simulink model "FAST_RL_Env"  (R2023a)
settings: Solver=FixedStepAuto  StartTime=0.0  StopTime=inf  FixedStep=DT  MaxStep=DT  RelTol=1e-3  EnableMultiTasking=on
undefined symbols (not defined in the file): Cmoment, Cpitch, MaxMoment, Penalty
libraries: rllib x1
settings Model: Creator=bjonkman  LastModifiedBy=Admin
settings SolverCC: AlgebraicLoopSolver=TrustRegion  AutoInsertRateTranBlk=on
settings DataIOCC: LimitDataPoints=on  SaveFormat=Array  SignalLoggingSaveFormat=ModelDataLogs  SaveOutput=off  SaveTime=off  SignalLoggingName=sigsOut
settings OptimizationCC: ReuseModelBlockBuffer=off  ExpressionDepthLimit=2147483647  LifeSpan=inf
settings DebuggingCC: SaveWithParameterizedLinksMsg=none  UnderspecifiedInitializationDetection=Classic  MergeDetectMultiDrivingBlocksExec=none  SignalResolutionControl=TryResolveAllWithWarning  MultiTaskDSMMsg=warning  MultiTaskCondExecSysMsg=none  FcnCallInpInsideContextMsg=warning  UnconnectedInputMsg=warning  UnconnectedOutputMsg=warning  UnconnectedLineMsg=warning  StateNameClashWarn=warning  SFUnexpectedBacktrackingDiag=warning  SFNoUnconditionalDefaultTransitionDiag=warning  SFExecutionAtInitializationDiag=none  ArithmeticOperatorsInVariantConditions=warning
settings HardwareCC: ProdBitPerPointer=32  ProdBitPerSizeT=32  ProdBitPerPtrDiffT=32  ProdLargestAtomicFloat=None  ProdIntDivRoundTo=Undefined  ProdEndianess=Unspecified  ProdWordSize=32  ProdHWDeviceType=32-bit Generic  TargetUnknown=on
settings ModelReferenceCC: EnableRefExpFcnMdlSchedulingChecks=on  PropagateSignalLabelsOutOfModel=off
settings SFSimCC: SimUseLocalCustomCode=off  CustomCodeUndefinedFunction=UseInterfaceOnly
settings RTWCC: RTWUseLocalCustomCode=off  DLArmComputeVersion=19.05
settings CodeAppCC: StateflowObjectComments=on
settings GRTTargetCC: TargetLangStandard=C89/C90 (ANSI)  CombineOutputUpdateFcns=off  GRTInterface=on
settings ConfigComp: CovMetricSettings=dw  CovSaveCumulativeToWorkspaceVar=on  CovSaveSingleToWorkspaceVar=on  CovExternalEMLEnable=off

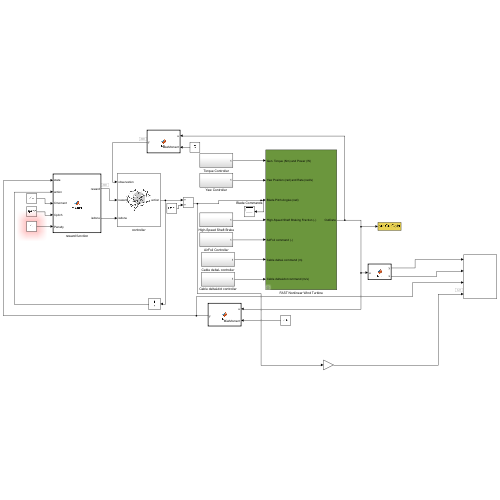
[thumbnail: Simulink's stored preview of the top-level diagram]
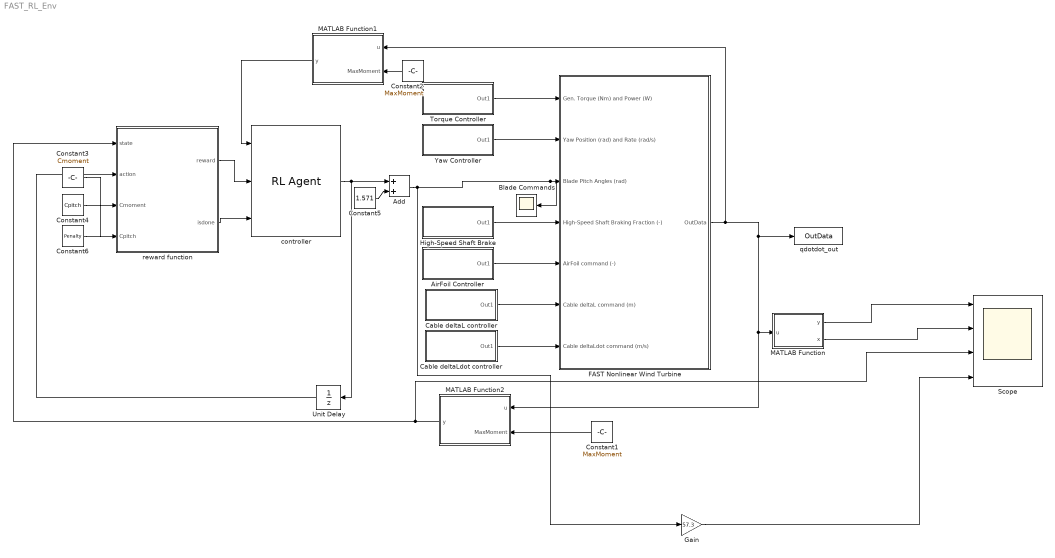
== system FAST_RL_Env ==
  Add : Sum
  AirFoil Controller : Subsystem
  Blade Commands : Scope
  Cable deltaL controller : Subsystem
  Cable deltaLdot controller : Subsystem
  Constant1 : Constant  Value=MaxMoment
  Constant2 : Constant  Value=MaxMoment
  Constant3 : Constant  Value=Cmoment
  Constant4 : Constant  Value=Cpitch
  Constant5 : Constant  Value=1.571
  Constant6 : Constant  Value=Penalty
  FAST Nonlinear Wind Turbine : Subsystem  mask(FAST Nonlinear Wind Turbine){}
      mask help: This block contains the FAST S-Function.
      mask init:
      | clear FAST_SFunc
  Gain : Gain  Gain=57.3
  High-Speed Shaft Brake : Subsystem
  MATLAB Function : MATLAB Function  TreatAsAtomicUnit=on
  MATLAB Function1 : MATLAB Function  TreatAsAtomicUnit=on
  MATLAB Function2 : MATLAB Function  TreatAsAtomicUnit=on
  Scope : Scope  NumInputPorts=4
  Torque Controller : Subsystem
  Unit Delay : UnitDelay  SampleTime=-1  HasFrameUpgradeWarning=on
  Yaw Controller : Subsystem
  controller : rllib/RL Agent  Agent=agent  ExternalActionAsInput=off  ProvideLastAction=off  ProvideCumRwd=off  TreatAsDirectFeedthrough=on  UseStrictObservationDataTypes=off
  qdotdot_out : ToWorkspace  VariableName=OutData  SampleTime=-1
  reward function : MATLAB Function  TreatAsAtomicUnit=on
  wires:
  Torque Controller/1(Out1) -> FAST Nonlinear Wind Turbine/1(Gen. Torque (Nm) and Power (W))
  Yaw Controller/1(Out1) -> FAST Nonlinear Wind Turbine/2(Yaw Position (rad) and Rate (rad/s))
  High-Speed Shaft Brake/1(Out1) -> FAST Nonlinear Wind Turbine/4(High-Speed Shaft Braking Fraction (-))
  AirFoil Controller/1(Out1) -> FAST Nonlinear Wind Turbine/5(AirFoil command (-))
  reward function/1(reward) -> controller/2
  Unit Delay/1 -> reward function/2(action)
  MATLAB Function/1(y) -> Scope/1
  MATLAB Function/2(x) -> Scope/2
  Cable deltaL controller/1(Out1) -> FAST Nonlinear Wind Turbine/6(Cable deltaL command (m))
  Cable deltaLdot controller/1(Out1) -> FAST Nonlinear Wind Turbine/7(Cable deltaLdot command (m/s))
  FAST Nonlinear Wind Turbine/1(OutData) -> MATLAB Function1/1(u), qdotdot_out/1, MATLAB Function2/1(u), MATLAB Function/1(u)
  MATLAB Function2/1(y) -> Scope/3, reward function/1(state)
  MATLAB Function1/1(y) -> controller/1
  controller/1 -> Add/1, Unit Delay/1
  Constant1/1 -> MATLAB Function2/2(MaxMoment)
  Constant2/1 -> MATLAB Function1/2(MaxMoment)
  Constant4/1 -> reward function/4(Cpitch)
  Constant3/1 -> reward function/3(Cmoment)
  Constant5/1 -> Add/2
  Gain/1 -> Scope/4
  Add/1 -> Blade Commands/1, FAST Nonlinear Wind Turbine/3(Blade Pitch Angles (rad)), Gain/1
  reward function/2(isdone) -> controller/3
  Constant6/1 -> ?

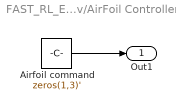
== system FAST_RL_Env/AirFoil Controller ==
  Airfoil command : Constant  Value=zeros(1,3)'
  Out1 : Outport
  wires:
  Airfoil command/1 -> Out1/1

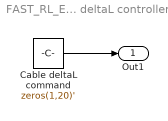
== system FAST_RL_Env/Cable deltaL controller ==
  Cable deltaL command : Constant  Value=zeros(1,20)'
  Out1 : Outport
  wires:
  Cable deltaL command/1 -> Out1/1

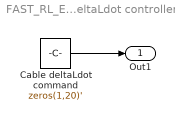
== system FAST_RL_Env/Cable deltaLdot controller ==
  Cable deltaLdot command : Constant  Value=zeros(1,20)'
  Out1 : Outport
  wires:
  Cable deltaLdot command/1 -> Out1/1

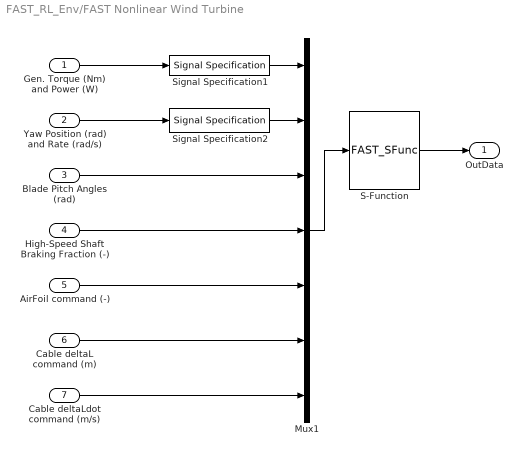
== system FAST_RL_Env/FAST Nonlinear Wind Turbine ==
  Gen. Torque (Nm) and Power (W) : Inport
  Yaw Position (rad) and Rate (rad/s) : Inport  Port=2
  Blade Pitch Angles (rad) : Inport  Port=3
  High-Speed Shaft Braking Fraction (-) : Inport  Port=4
  AirFoil command (-) : Inport  Port=5
  Cable deltaL command (m) : Inport  Port=6
  Cable deltaLdot command (m/s) : Inport  Port=7
  Mux1 : Mux  Inputs=7
  S-Function : S-Function  FunctionName=FAST_SFunc  Parameters=FAST_InputFileName, TMax, 0  SFunctionDeploymentMode=off  EnableBusSupport=off
  Signal Specification1 : SignalSpecification  OutDataTypeStr=double  Dimensions=2
  Signal Specification2 : SignalSpecification  OutDataTypeStr=double  Dimensions=2
  OutData : Outport
  wires:
  Gen. Torque (Nm) and Power (W)/1 -> Signal Specification1/1
  S-Function/1 -> OutData/1
  Mux1/1 -> S-Function/1
  Blade Pitch Angles (rad)/1 -> Mux1/3
  Yaw Position (rad) and Rate (rad/s)/1 -> Signal Specification2/1
  Signal Specification1/1 -> Mux1/1
  Signal Specification2/1 -> Mux1/2
  High-Speed Shaft Braking Fraction (-)/1 -> Mux1/4
  AirFoil command (-)/1 -> Mux1/5
  Cable deltaL command (m)/1 -> Mux1/6
  Cable deltaLdot command (m/s)/1 -> Mux1/7

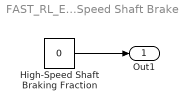
== system FAST_RL_Env/High-Speed Shaft Brake ==
  High-Speed Shaft Braking Fraction : Constant  Value=0
  Out1 : Outport
  wires:
  High-Speed Shaft Braking Fraction/1 -> Out1/1

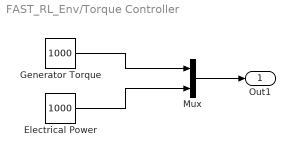
== system FAST_RL_Env/Torque Controller ==
  Electrical Power : Constant  Value=1000
  Generator Torque : Constant  Value=1000
  Mux : Mux  Inputs=2
  Out1 : Outport
  wires:
  Mux/1 -> Out1/1
  Generator Torque/1 -> Mux/1
  Electrical Power/1 -> Mux/2

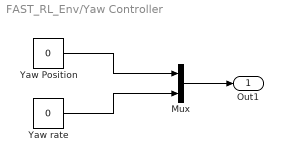
== system FAST_RL_Env/Yaw Controller ==
  Mux : Mux  Inputs=2
  Yaw Position : Constant  Value=0
  Yaw rate : Constant  Value=0
  Out1 : Outport
  wires:
  Mux/1 -> Out1/1
  Yaw Position/1 -> Mux/1
  Yaw rate/1 -> Mux/2

== matlab function FAST_RL_Env/MATLAB Function ==
  data: u input; y output; x output
function [y,x] = fcn(u)

y = u(18,:); %Heave
x = u(19,:); %Pitch

== matlab function FAST_RL_Env/reward function ==
  data: state input; action input; reward output; Cmoment input; Cpitch input; isdone output
function [reward,isdone]   = reward(state, action, Cmoment,Cpitch)

%roll = state(18)/;
%pitch = state(16);
%surge = state(12);
%sway = state(16);
%heave = state(14);

%basemoment = state(36);
%power = state(39)/100000;
rollMoment = state(1) ;
pitchMoment = state(2) ;
yawMoment = state(3) ;


%moveLine1 = action(1);

reward = -Cmoment*rollMoment^2 - Cmoment*pitchMoment^2 - Cmoment*rollMoment^2 - Cpitch*action(1)^2 - Cpitch*action(2)^2 - Cpitch*action(3)^2;
% if abs(rollMoment) > 1 || abs(pitchMoment) > 1 || abs(yawMoment) > 1 
%     isdone = true ;
%     reward = reward - Penalty ;
% else
%     isdone = false;
% end

== matlab function FAST_RL_Env/MATLAB Function1 ==
  data: u input; y output; MaxMoment input
function y  = fcn(u,MaxMoment)

y = [u(2,:) , u(39,:)/MaxMoment, u(40,:)/MaxMoment, u(41,:)/MaxMoment] ; %Heave

== matlab function FAST_RL_Env/MATLAB Function2 ==
  data: u input; y output; MaxMoment input
function y  = fcn(u,MaxMoment)

y = [u(39,:)/MaxMoment, u(40,:)/MaxMoment, u(41,:)/MaxMoment] ; %Heave
